simulink model "Pendulum"  (R2018a)
settings: Solver=ode45  StartTime=tmin  StopTime=tmax  RelTol=1e-3
values from neighbouring files (symbols this model uses):
  g = 9.81    [L13T1_Pendulum.m]
  l = [ 1 1 ]    [L13T1_Pendulum.m]
  m = [ 1 1 ]    [L13T1_Pendulum.m]
  theta0 = [ deg2rad(90) deg2rad(-90) deg2rad(50) 0]    [L13T1_Pendulum.m]
settings Model: Creator=meron  LastModifiedBy=meron
settings HardwareCC: ProdHWDeviceType=AMD->x86-64 (Windows64)
settings RTWCC: TargetLang=C++
settings GRTTargetCC: TargetLangStandard=C++03 (ISO)  MultiInstanceERTCode=on  CodeInterfacePackaging=C++ class

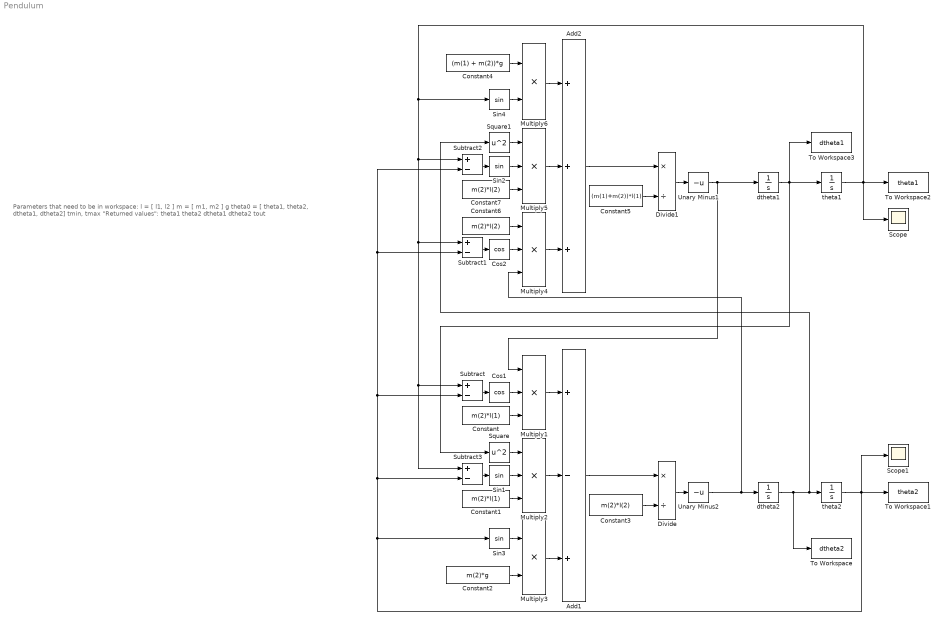
== system Pendulum ==
  note: Parameters that need to be in workspace:
      | l = [ l1, l2 ]
      | m = [ m1, m2 ]
      | g
      | theta0 = [ theta1, theta2, dtheta1, dtheta2]
      | tmin, tmax
      |
      | "Returned values":
      | theta1
      | theta2
      | dtheta1
      | dtheta2
      | tout
  Add1 : Sum  Inputs=+-+
  Add2 : Sum  Inputs=+++
  Constant : Constant  Value=m(2)*l(1)
  Constant1 : Constant  Value=m(2)*l(1)
  Constant2 : Constant  Value=m(2)*g
  Constant3 : Constant  Value=m(2)*l(2)
  Constant4 : Constant  Value=(m(1) + m(2))*g
  Constant5 : Constant  Value=(m(1)+m(2))*l(1)
  Constant6 : Constant  Value=m(2)*l(2)
  Constant7 : Constant  Value=m(2)*l(2)
  Cos1 : Trigonometry  Operator=cos
  Cos2 : Trigonometry  Operator=cos
  Divide : Product  Inputs=*/
  Divide1 : Product  Inputs=*/
  Multiply{1..2,4..5} (4 alike) : Product  Inputs=3
  Multiply3 : Product
  Multiply6 : Product
  Scope : Scope
  Scope1 : Scope
  Sin{1..4} (4 alike) : Trigonometry
  Square : Math  Operator=square  SaturateOnIntegerOverflow=on
  Square1 : Math  Operator=square  SaturateOnIntegerOverflow=on
  Subtract{,1..3} (4 alike) : Sum  Inputs=+-
  To Workspace : ToWorkspace  VariableName=dtheta2  SampleTime=-1
  To Workspace1 : ToWorkspace  VariableName=theta2  SampleTime=-1
  To Workspace2 : ToWorkspace  VariableName=theta1  SampleTime=-1
  To Workspace3 : ToWorkspace  VariableName=dtheta1  SampleTime=-1
  Unary Minus1 : UnaryMinus
  Unary Minus2 : UnaryMinus
  dtheta1 : Integrator  InitialCondition=theta0(3)
  dtheta2 : Integrator  InitialCondition=theta0(4)
  theta1 : Integrator  InitialCondition=theta0(1)
  theta2 : Integrator  InitialCondition=theta0(2)
  wires:
  Constant/1 -> Multiply1/3
  Cos1/1 -> Multiply1/2
  Multiply2/1 -> Add1/2
  Constant1/1 -> Multiply2/3
  Sin1/1 -> Multiply2/2
  Square/1 -> Multiply2/1
  Constant2/1 -> Multiply3/2
  Add1/1 -> Divide/1
  Constant3/1 -> Divide/2
  Divide/1 -> Unary Minus2/1
  Unary Minus2/1 -> dtheta2/1, Multiply4/3
  dtheta2/1 -> To Workspace/1, Square1/1, theta2/1
  Multiply6/1 -> Add2/1
  Multiply4/1 -> Add2/3
  Add2/1 -> Divide1/1
  Multiply5/1 -> Add2/2
  Sin2/1 -> Multiply5/2
  dtheta1/1 -> To Workspace3/1, theta1/1, Square/1
  Divide1/1 -> Unary Minus1/1
  Cos2/1 -> Multiply4/2
  Unary Minus1/1 -> dtheta1/1, Multiply1/1
  Square1/1 -> Multiply5/1
  Sin3/1 -> Multiply3/1
  Multiply3/1 -> Add1/3
  Multiply1/1 -> Add1/1
  Subtract/1 -> Cos1/1
  Subtract1/1 -> Cos2/1
  Subtract2/1 -> Sin2/1
  Subtract3/1 -> Sin1/1
  Sin4/1 -> Multiply6/2
  Constant4/1 -> Multiply6/1
  Constant5/1 -> Divide1/2
  Constant6/1 -> Multiply4/1
  Constant7/1 -> Multiply5/3
  theta1/1 -> Scope/1, To Workspace2/1, Sin4/1, Subtract2/1, Subtract/1, Subtract3/1, Subtract1/1
  theta2/1 -> Scope1/1, To Workspace1/1, Sin3/1, Subtract3/2, Subtract/2, Subtract1/2, Subtract2/2
